simulink model "Stabilisation_trajectoire_variable"  (R2018a)
settings: Solver=ode45  StartTime=0.0  StopTime=60.0  RelTol=1e-3  EnableMultiTasking=on
settings Model: Creator=Dalil  LastModifiedBy=dalil
settings DataIOCC: LimitDataPoints=on  SaveFormat=Array
settings OptimizationCC: ExpressionDepthLimit=2147483647  LifeSpan=inf
settings DebuggingCC: UnderspecifiedInitializationDetection=Classic  MergeDetectMultiDrivingBlocksExec=none  SolverPrmCheckMsg=warning  StateNameClashWarn=warning  SFUnexpectedBacktrackingDiag=warning  SFNoUnconditionalDefaultTransitionDiag=warning  SFExecutionAtInitializationDiag=none
settings HardwareCC: ProdBitPerPointer=32  ProdBitPerSizeT=32  ProdBitPerPtrDiffT=32  ProdLargestAtomicFloat=None  ProdIntDivRoundTo=Undefined  ProdEndianess=Unspecified  ProdWordSize=32  ProdHWDeviceType=32-bit Generic
settings ModelReferenceCC: PropagateSignalLabelsOutOfModel=off
settings CodeAppCC: StateflowObjectComments=on
settings GRTTargetCC: TargetLangStandard=C89/C90 (ANSI)  GeneratePreprocessorConditionals=Disable all
settings ConfigComp: CovMetricSettings=dw  CovHtmlReporting=on  CovSaveCumulativeToWorkspaceVar=on  CovSaveSingleToWorkspaceVar=on  CovExternalEMLEnable=off

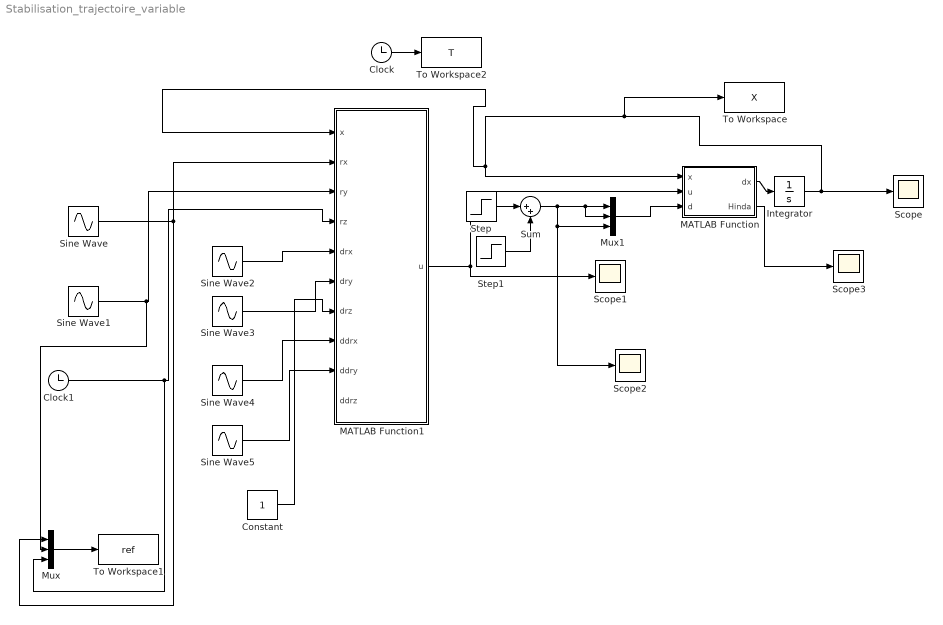
== system Stabilisation_trajectoire_variable ==
  Clock : Clock
  Clock1 : Clock
  Constant : Constant
  Integrator : Integrator  InitialCondition=0.1*[1 1 1 1 1 1 1 1 1 1 1 1]
  MATLAB Function : MATLAB Function  TreatAsAtomicUnit=on
  MATLAB Function1 : MATLAB Function  TreatAsAtomicUnit=on
  Mux : Mux  Inputs=3
  Mux1 : Mux  Inputs=3
  Scope{,1..3} (4 alike) : Scope
  Sine Wave : Sin  SampleTime=0
  Sine Wave1 : Sin  Phase=pi/2  SampleTime=0
  Sine Wave2 : Sin  Phase=pi/2  SampleTime=0
  Sine Wave3 : Sin  Amplitude=-1  SampleTime=0
  Sine Wave4 : Sin  Amplitude=-1  SampleTime=0
  Sine Wave5 : Sin  Amplitude=-1  Phase=pi/2  SampleTime=0
  Step : Step  Time=30  SampleTime=0
  Step1 : Step  Time=33  After=-1  SampleTime=0
  Sum : Sum  Inputs=|++
  To Workspace : ToWorkspace  VariableName=X  SampleTime=-1
  To Workspace1 : ToWorkspace  VariableName=ref  SampleTime=-1
  To Workspace2 : ToWorkspace  VariableName=T  SampleTime=-1
  wires:
  MATLAB Function/1(dx) -> Integrator/1
  Integrator/1 -> To Workspace/1, MATLAB Function/1(x), MATLAB Function1/1(x), Scope/1
  MATLAB Function1/1(u) -> Scope1/1, MATLAB Function/2(u)
  Sine Wave/1 -> Mux/1, MATLAB Function1/2(rx)
  Sine Wave1/1 -> Mux/2, MATLAB Function1/3(ry)
  Clock1/1 -> Mux/3, MATLAB Function1/4(rz)
  Mux/1 -> To Workspace1/1
  Clock/1 -> To Workspace2/1
  Sine Wave2/1 -> MATLAB Function1/5(drx)
  Sine Wave3/1 -> MATLAB Function1/6(dry)
  Sine Wave4/1 -> MATLAB Function1/8(ddrx)
  Sine Wave5/1 -> MATLAB Function1/9(ddry)
  Constant/1 -> MATLAB Function1/7(drz)
  Mux1/1 -> MATLAB Function/3(d)
  Step/1 -> Sum/1
  Step1/1 -> Sum/2
  Sum/1 -> Scope2/1, Mux1/3, Mux1/2, Mux1/1
  MATLAB Function/2(Hinda) -> Scope3/1

== matlab function Stabilisation_trajectoire_variable/MATLAB Function1 ==
  data: x input; u output; rx input; ry input; rz input; drx input; dry input; drz input; ddrx input; ddry input; ddrz input
function u = fcn(x,rx,ry,rz,drx,dry,drz,ddrx,ddry,ddrz)
%#codegen


u = zeros(6,1);

g  = 9.81;

% les moments inirtiels 
Ixx=7.5*10^-3;
Iyy=7.5*10^-3;
Izz=1.3*10^-3;

k1 = 2; k2 = 3;
k3 = 3; k4 = 5;
k5 = 2; k6 = 4;
k7 = 2; k8 = 3;
k9 = 2; k10 = 6;
k11 = 2; k12 = 3;

% les coeficients 
a1=((Iyy-Izz)/Ixx);
a2=((Izz-Ixx)/Iyy);
a3=((Ixx-Iyy)/Izz);

% Commande classique poursuite de trajectoire
u(1) = -(x(12)*x(4)-x(10)*x(6)-g*sin(x(9)))-k1*(x(1)-rx)-k2*(x(2)-drx)+ddrx;
u(2) = -(x(8)*x(6)-x(12)*x(2)+g*sin(x(7))*cos(x(9)))-k3*(x(3)-ry)-k4*(x(4)-dry)+ddry;
u(3) = -(x(10)*x(2)-x(8)*x(4)+g*cos(x(7))*cos(x(9)))-k5*(x(5)-rz)-k6*(x(6)-drz)+ddrz;
u(4) = -(a1*x(12)*x(10))-k7*x(7)-k8*x(8);
u(5) = -a2*x(12)*x(8)-k9*x(9)-k10*x(10);
u(6) = -a3*x(8)*x(10)-k11*x(11)-k12*x(12);

% commande modes glissants d'ordre 1
% u(1) = -k1*(x(1)-rx)-k2*(x(2)-drx)+ddrx-1*sign(x(1)-rx)-1*sign(x(2)-drx);
% u(2) = -k3*(x(3)-ry)-k4*(x(4)-dry)+ddry-1*sign(x(3)-ry)-1*sign(x(4)-dry);
% u(3) = -k5*(x(5)-rz)-k6*(x(6)-drz)+ddrz-2*sign(x(5)-rz)-2*sign(x(6)-drz);
% u(4) = -(a1*x(12)*x(10))-k7*x(7)-k8*x(8);
% u(5) = -a2*x(12)*x(8)-k9*x(9)-k10*x(10);
% u(6) = -a3*x(8)*x(10)-k11*x(11)-k12*x(12);

== matlab function Stabilisation_trajectoire_variable/MATLAB Function ==
  data: x input; u input; dx output; d input; Hinda output
function [dx,Hinda] = fcn(x,u,d)
%#codegen

g  = 9.81;

% les moments inirtiels 
Ixx=7.5*10^-3;
Iyy=7.5*10^-3;
Izz=1.3*10^-3;


% les coeficients 
a1=((Iyy-Izz)/Ixx);
a2=((Izz-Ixx)/Iyy);
a3=((Ixx-Iyy)/Izz);

dx = zeros(12,1);

dx(1) = x(2);
dx(2) = x(12)*x(4)-x(10)*x(6)-g*sin(x(9))+u(1)+d(1);
dx(3) = x(4);
dx(4) = x(8)*x(6)-x(12)*x(2)+g*sin(x(7))*cos(x(9))+u(2)+d(2);
dx(5) = x(6);
dx(6) = x(10)*x(2)-x(8)*x(4)+g*cos(x(7))*cos(x(9))+u(3)+d(3);
dx(7) = x(8);
dx(8) = a1*x(12)*x(10)+u(4);
dx(9) = x(10);
dx(10) = a2*x(12)*x(8)+u(5);
dx(11) = x(12);
dx(12) = a3*x(8)*x(10)+u(6);

Hinda = x(10)*x(2)-x(8)*x(4)+g*cos(x(7))*cos(x(9))+d(3);
